simulink model "simulinkReCompensated"  (R2015a)
settings: Solver=ode45  StartTime=0.0  StopTime=10.0  RelTol=1e-3
settings Model: Creator=theVenom  LastModifiedBy=theVenom

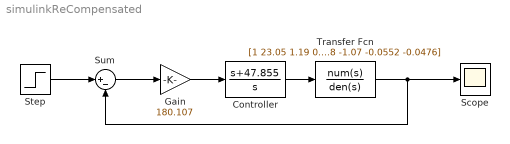
== system simulinkReCompensated ==
  Controller : TransferFcn  Numerator=[1 47.855]  Denominator=[1 0]
  Gain : Gain  Gain=180.107
  Scope : Scope
      settings: YMin=0.87821  YMax=1.4382
  Step : Step  SampleTime=0
  Sum : Sum  Inputs=|+-
  Transfer Fcn : TransferFcn  Numerator=[1 23.05 1.19 0.92]  Denominator=[1 1.08 -1.07 -0.0552 -0.0476]
  wires:
  Transfer Fcn/1 -> Sum/2, Scope/1
  Step/1 -> Sum/1
  Sum/1 -> Gain/1
  Gain/1 -> Controller/1
  Controller/1 -> Transfer Fcn/1
